simulink model "thrust_vector_rocket2_no_thrust"  (R2024b)
settings: Solver=VariableStepAuto  StartTime=0.0  StopTime=10  RelTol=1e-3
values from neighbouring files (symbols this model uses):
  A = [0 1; 0 0]    [model1_simplified.m]    (also in model2_no_thrustl.m = [0, 1, 0, 0, 0, 0; model3_thrust.m = [0, 1,      0, 0,       0, 0; model4_system_and_stability.m = jacobian(f, x))
  B = [0; -T*L/J]    [model1_simplified.m]    (also in model2_no_thrustl.m = [0; model3_thrust.m = [0   0; model4_system_and_stability.m = jacobian(f, u))
  C = [1 0]    [model1_simplified.m]    (also in model2_no_thrustl.m = [1 0 0 0 0 0; model3_thrust.m = [1 0 0 0 0 0; model4_system_and_stability.m = [1 0 0 0 0 0)
  D = 0    [model1_simplified.m]    (also in model2_no_thrustl.m = [0; 0; 0]; model3_thrust.m = [0 0; 0 0; 0 0]; model4_system_and_stability.m)
  reg = ss(A1, sys.b, sys.c, 0)    [model2_no_thrustl.m]    (also in model3_thrust.m)
  sys = ss(A,B,C,D)    [model1_simplified.m]    (also in model2_no_thrustl.m; model3_thrust.m; model4_system_and_stability.m = ss(A, B, eye(6), zeros(6,2)))
  Ts = 0.05    [model2_no_thrustl.m]    (also in model3_thrust.m; optimal_control.m; rocketParameters.mat)
  x0 = [0; 0; 0; 0; 5*pi/180; 0]    [model2_no_thrustl.m]    (also in model3_thrust.m)
libraries: slpidlib x4, mpclib x2
settings Model: Creator=wolfl  LastModifiedBy=wolfl

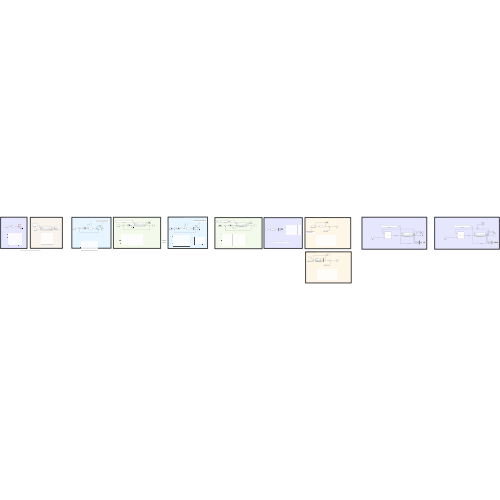
[thumbnail: Simulink's stored preview of the top-level diagram]
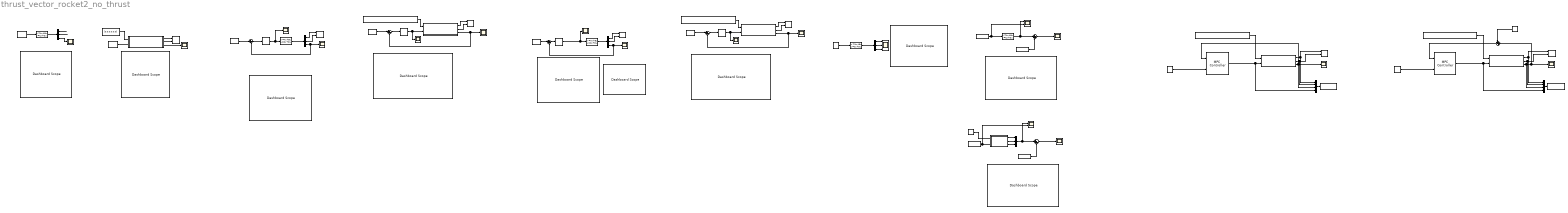
== system thrust_vector_rocket2_no_thrust ==
  note: ATTIVARE L'
      |
      | antiwindup
  note: Model Predictive Control
  note: NOTA: ricordati di selezionare "hold final value" nell'input, se no il sistema diverge malissimo!
  note: Optimal Control
  note: We can notice that this regulator allows the states to converge!
  note: Regulator with Pole Placement
  note: Non linear closed-loop
  note: Linear closed-loop
  note: Non linear open-loop
  note: Linear open-loop
  note: NOTE: We can see that in the linearized system,
      | the rocket doesn't loose altitude when it steers
  note: We can notice that the open.loop dynamic is similar only in the first few seconds.
  note: Non linear closed-loop
  note: Linear closed-loop with discrete-time controller
  note: NOTE: We can see that in the linearized system,
      | the rocket doesn't loose altitude when it steers
  note: Optimal Control - non linear system
  note: Model Predictive Control
  A+B*K : StateSpace  A=reg.a  B=reg.b  C=reg.c  D=reg.d  InitialCondition=[1,1,0,0,5*pi/180,0]
  Constant : Constant  Value=0
  Constant1 : Constant  Value=x0
  Dashboard Scope{,1..9} (10 alike) : DashboardScope
  Demux{,1..3} (4 alike) : Demux  Outputs=3
  Error : Scope
  Error1 : Scope
  Expected Output : FromWorkspace  VariableName=ySim
  Expected Output1 : FromWorkspace  VariableName=ySim
  Input from Optimal Control : FromWorkspace  VariableName=uSim  SampleTime=Ts  OutputAfterFinalValue=Holding final value
  Input from Optimal Control1 : FromWorkspace  VariableName=uSim  SampleTime=Ts  OutputAfterFinalValue=Holding final value
  MPC Controller : mpclib/MPC Controller  SCDEnableBlockLinearizationSpecification=on  mpcobj=mpc1  is_multiple=0  enable_value=0  return_u0=off  updateMPCinCallerWorkspace=on  md_inport=off  mv_inport=off  uref_inport=off  return_cost=off  return_mvseq=off  return_qpstatus=off  return_xseq=off  return_state=off  return_ovseq=off  state_inport=off  umin_inport=off  umax_inport=off  ymin_inport=off  ymax_inport=off  cc_inport=off  ywt_inport=off  uwt_inport=off  duwt_inport=off  rhoeps_inport=off  pm_inport=off  MaximumP=10  HorizonChoice=FixedHorizon  n_ts=0.05  n_p=10  n_mv=1  n_md=0  n_ud=0  n_mo=1  n_uo=0  BlockDataType=double  SampleTimeInherited=off  switch_inport=off
  MPC Controller1 : mpclib/MPC Controller  SCDEnableBlockLinearizationSpecification=on  mpcobj=mpc1  is_multiple=0  enable_value=0  return_u0=off  updateMPCinCallerWorkspace=on  md_inport=off  mv_inport=off  uref_inport=off  return_cost=off  return_mvseq=off  return_qpstatus=off  return_xseq=off  return_state=off  return_ovseq=off  state_inport=off  umin_inport=off  umax_inport=off  ymin_inport=off  ymax_inport=off  cc_inport=off  ywt_inport=off  uwt_inport=off  duwt_inport=off  rhoeps_inport=off  pm_inport=off  MaximumP=10  HorizonChoice=FixedHorizon  n_ts=0.05  n_p=10  n_mv=1  n_md=0  n_ud=0  n_mo=1  n_uo=0  BlockDataType=double  SampleTimeInherited=off  switch_inport=off
  Mux : Mux  Inputs=3
  Mux1 : Mux
  Mux2 : Mux
  Non linear System : Subsystem
  Non linear System1 : Subsystem
  Non linear System2 : Subsystem
  Non linear System3 : Subsystem
  PID Controller : slpidlib/PID Controller  Controller=PID  Form=Parallel  TimeDomain=Continuous-time  UseExternalTs=off  SampleTime=-1  IntegratorMethod=Forward Euler  FilterMethod=Forward Euler  ControllerParametersSource=internal  P=-0.206944152604434  I=-0.0701836790588113  UseKiTs=off  D=-0.149835070791128  UseExternalDerivativeSource=off  N=39.5105217733355  UseFilter=on  TunerSelectOption=Transfer Function Based (PID Tuner App)  InitialConditionSource=internal  InitialConditionForIntegrator=0  InitialConditionForFilter=0  DifferentiatorICPrevScaledInput=0  ExternalReset=none  TrackingMode=off  Kt=1  LimitOutput=on  SatLimitsSource=internal  UpperSaturationLimit=30*pi/180  LowerSaturationLimit=-30*pi/180  LinearizeAsGain=on  AntiWindupMode=none  Kb=1  LimitIntegrator=off  UpperIntegratorSaturationLimit=inf  LowerIntegratorSaturationLimit=-inf  POutMin=[]  POutMax=[]  IOutMin=[]  IOutMax=[]  DOutMin=[]  DOutMax=[]  NOutMin=[]  NOutMax=[]  SumOutMin=[]  SumOutMax=[]  SaturationOutMin=[]  SaturationOutMax=[]  PParamMin=[]  PParamMax=[]  IParamMin=[]  IParamMax=[]  DParamMin=[]  DParamMax=[]  NParamMin=[]  NParamMax=[]  KbParamMin=[]  KbParamMax=[]  KtParamMin=[]  KtParamMax=[]  KbOutMin=[]  KbOutMax=[]  KtOutMin=[]  KtOutMax=[]  IntegratorOutMin=[]  IntegratorOutMax=[]  FilterOutMin=[]  FilterOutMax=[]  SumI1OutMin=[]  SumI1OutMax=[]  SumI2OutMin=[]  SumI2OutMax=[]  SumI3OutMin=[]  SumI3OutMax=[]  SumI4OutMin=[]  SumI4OutMax=[]  SumDOutMin=[]  SumDOutMax=[]  DifferentiatorOutMin=[]  DifferentiatorOutMax=[]  FilterDiffOutCoefMin=[]  FilterDiffOutCoefMax=[]  ReciprocalOutMin=[]  ReciprocalOutMax=[]  SumDenOutMin=[]  SumDenOutMax=[]  SumNumOutMin=[]  SumNumOutMax=[]  DivideOutMin=[]  DivideOutMax=[]  UdiffTsProdOutMin=[]  UdiffTsProdOutMax=[]  NTsProdOutMin=[]  NTsProdOutMax=[]  UintegralTsProdOutMin=[]  UintegralTsProdOutMax=[]  UngainTsProdOutMin=[]  UngainTsProdOutMax=[]  ClampingZeroOutDataTypeStr=Inherit: Inherit via back propagation  ClampingZeroOutMin=[]  ClampingZeroOutMax=[]  FilterDenConstantOutDataTypeStr=Inherit: Inherit via back propagation  FilterDenConstantOutMin=[]  FilterDenConstantOutMax=[]  PCopyOutDataTypeStr=Inherit: Inherit via back propagation  PCopyOutMin=[]  PCopyOutMax=[]  NCopyOutDataTypeStr=Inherit: Inherit via back propagation  NCopyOutMin=[]  NCopyOutMax=[]  IntegratorContinuousStateAttributes=''  IntegratorStateMustResolveToSignalObject=off  IntegratorRTWStateStorageClass=Auto  FilterContinuousStateAttributes=''  FilterStateMustResolveToSignalObject=off  FilterRTWStateStorageClass=Auto  ParallelPVariant=InternalParameters  IdealPVariant=Disabled  IVariant=InternalParameters  DVariant=InternalParameters  IntegratorVariant=Continuous  SatVariant=Enabled  AWVariant=Passthrough  PCopyVariant=Disabled  TRVariant=Disabled  FdbkBlocksVariant=Forward  IdealPFdbkVariant=Disabled  SatFdbkVariant=Disabled  DerivativeFilterVariant=ContFilter  NVariant=InternalParameters  NCopyVariant=Disabled  FilterICVariant=InternalICsFilter  IntegratorICVariant=InternalICs  ExternalResetVariant=Disabled  TRSumVariant=Passthrough  SumFdbkVariant=Disabled  SumVariant=Sum_PID  TsampFilterVariant=InternalTs  TsampNgainVariant=Passthrough  TsampIntegralVariant=Disabled_SignalSpec  ExternalSaturationOutDataTypeStr=Inherit: Same as second input  DerivativeSourceVariant=ErrorSignal  PreIntVariant=InternalPreInt
  PID Controller1 : slpidlib/PID Controller  Controller=PID  Form=Parallel  TimeDomain=Continuous-time  UseExternalTs=off  SampleTime=-1  IntegratorMethod=Forward Euler  FilterMethod=Forward Euler  ControllerParametersSource=internal  P=-0.206944152604434  I=-0.0701836790588113  UseKiTs=off  D=-0.149835070791128  UseExternalDerivativeSource=off  N=39.5105217733355  UseFilter=on  TunerSelectOption=Transfer Function Based (PID Tuner App)  InitialConditionSource=internal  InitialConditionForIntegrator=0  InitialConditionForFilter=0  DifferentiatorICPrevScaledInput=0  ExternalReset=none  TrackingMode=off  Kt=1  LimitOutput=on  SatLimitsSource=internal  UpperSaturationLimit=30*pi/180  LowerSaturationLimit=-30*pi/180  LinearizeAsGain=on  AntiWindupMode=none  Kb=1  LimitIntegrator=off  UpperIntegratorSaturationLimit=inf  LowerIntegratorSaturationLimit=-inf  POutMin=[]  POutMax=[]  IOutMin=[]  IOutMax=[]  DOutMin=[]  DOutMax=[]  NOutMin=[]  NOutMax=[]  SumOutMin=[]  SumOutMax=[]  SaturationOutMin=[]  SaturationOutMax=[]  PParamMin=[]  PParamMax=[]  IParamMin=[]  IParamMax=[]  DParamMin=[]  DParamMax=[]  NParamMin=[]  NParamMax=[]  KbParamMin=[]  KbParamMax=[]  KtParamMin=[]  KtParamMax=[]  KbOutMin=[]  KbOutMax=[]  KtOutMin=[]  KtOutMax=[]  IntegratorOutMin=[]  IntegratorOutMax=[]  FilterOutMin=[]  FilterOutMax=[]  SumI1OutMin=[]  SumI1OutMax=[]  SumI2OutMin=[]  SumI2OutMax=[]  SumI3OutMin=[]  SumI3OutMax=[]  SumI4OutMin=[]  SumI4OutMax=[]  SumDOutMin=[]  SumDOutMax=[]  DifferentiatorOutMin=[]  DifferentiatorOutMax=[]  FilterDiffOutCoefMin=[]  FilterDiffOutCoefMax=[]  ReciprocalOutMin=[]  ReciprocalOutMax=[]  SumDenOutMin=[]  SumDenOutMax=[]  SumNumOutMin=[]  SumNumOutMax=[]  DivideOutMin=[]  DivideOutMax=[]  UdiffTsProdOutMin=[]  UdiffTsProdOutMax=[]  NTsProdOutMin=[]  NTsProdOutMax=[]  UintegralTsProdOutMin=[]  UintegralTsProdOutMax=[]  UngainTsProdOutMin=[]  UngainTsProdOutMax=[]  ClampingZeroOutDataTypeStr=Inherit: Inherit via back propagation  ClampingZeroOutMin=[]  ClampingZeroOutMax=[]  FilterDenConstantOutDataTypeStr=Inherit: Inherit via back propagation  FilterDenConstantOutMin=[]  FilterDenConstantOutMax=[]  PCopyOutDataTypeStr=Inherit: Inherit via back propagation  PCopyOutMin=[]  PCopyOutMax=[]  NCopyOutDataTypeStr=Inherit: Inherit via back propagation  NCopyOutMin=[]  NCopyOutMax=[]  IntegratorContinuousStateAttributes=''  IntegratorStateMustResolveToSignalObject=off  IntegratorRTWStateStorageClass=Auto  FilterContinuousStateAttributes=''  FilterStateMustResolveToSignalObject=off  FilterRTWStateStorageClass=Auto  ParallelPVariant=InternalParameters  IdealPVariant=Disabled  IVariant=InternalParameters  DVariant=InternalParameters  IntegratorVariant=Continuous  SatVariant=Enabled  AWVariant=Passthrough  PCopyVariant=Disabled  TRVariant=Disabled  FdbkBlocksVariant=Forward  IdealPFdbkVariant=Disabled  SatFdbkVariant=Disabled  DerivativeFilterVariant=ContFilter  NVariant=InternalParameters  NCopyVariant=Disabled  FilterICVariant=InternalICsFilter  IntegratorICVariant=InternalICs  ExternalResetVariant=Disabled  TRSumVariant=Passthrough  SumFdbkVariant=Disabled  SumVariant=Sum_PID  TsampFilterVariant=InternalTs  TsampNgainVariant=Passthrough  TsampIntegralVariant=Disabled_SignalSpec  ExternalSaturationOutDataTypeStr=Inherit: Same as second input  DerivativeSourceVariant=ErrorSignal  PreIntVariant=InternalPreInt
  PID Controller2 : slpidlib/PID Controller  Controller=PID  Form=Parallel  TimeDomain=Discrete-time  UseExternalTs=off  SampleTime=0.1  IntegratorMethod=Forward Euler  FilterMethod=Forward Euler  ControllerParametersSource=internal  P=-0.000166400925594158  I=-1.78058545909458e-06  UseKiTs=off  D=-0.0038876634505011  UseExternalDerivativeSource=off  N=1.14439525064094  UseFilter=off  TunerSelectOption=Transfer Function Based (PID Tuner App)  InitialConditionSource=internal  InitialConditionForIntegrator=0  InitialConditionForFilter=0  DifferentiatorICPrevScaledInput=0  ExternalReset=none  TrackingMode=off  Kt=1  LimitOutput=on  SatLimitsSource=internal  UpperSaturationLimit=30*pi/180  LowerSaturationLimit=-30*pi/180  LinearizeAsGain=on  AntiWindupMode=none  Kb=1  LimitIntegrator=off  UpperIntegratorSaturationLimit=inf  LowerIntegratorSaturationLimit=-inf  POutMin=[]  POutMax=[]  IOutMin=[]  IOutMax=[]  DOutMin=[]  DOutMax=[]  NOutMin=[]  NOutMax=[]  SumOutMin=[]  SumOutMax=[]  SaturationOutMin=[]  SaturationOutMax=[]  PParamMin=[]  PParamMax=[]  IParamMin=[]  IParamMax=[]  DParamMin=[]  DParamMax=[]  NParamMin=[]  NParamMax=[]  KbParamMin=[]  KbParamMax=[]  KtParamMin=[]  KtParamMax=[]  KbOutMin=[]  KbOutMax=[]  KtOutMin=[]  KtOutMax=[]  IntegratorOutMin=[]  IntegratorOutMax=[]  FilterOutMin=[]  FilterOutMax=[]  SumI1OutMin=[]  SumI1OutMax=[]  SumI2OutMin=[]  SumI2OutMax=[]  SumI3OutMin=[]  SumI3OutMax=[]  SumI4OutMin=[]  SumI4OutMax=[]  SumDOutMin=[]  SumDOutMax=[]  DifferentiatorOutMin=[]  DifferentiatorOutMax=[]  FilterDiffOutCoefMin=[]  FilterDiffOutCoefMax=[]  ReciprocalOutMin=[]  ReciprocalOutMax=[]  SumDenOutMin=[]  SumDenOutMax=[]  SumNumOutMin=[]  SumNumOutMax=[]  DivideOutMin=[]  DivideOutMax=[]  UdiffTsProdOutMin=[]  UdiffTsProdOutMax=[]  NTsProdOutMin=[]  NTsProdOutMax=[]  UintegralTsProdOutMin=[]  UintegralTsProdOutMax=[]  UngainTsProdOutMin=[]  UngainTsProdOutMax=[]  ClampingZeroOutDataTypeStr=Inherit: Inherit via back propagation  ClampingZeroOutMin=[]  ClampingZeroOutMax=[]  FilterDenConstantOutDataTypeStr=Inherit: Inherit via back propagation  FilterDenConstantOutMin=[]  FilterDenConstantOutMax=[]  PCopyOutDataTypeStr=Inherit: Inherit via back propagation  PCopyOutMin=[]  PCopyOutMax=[]  NCopyOutDataTypeStr=Inherit: Inherit via back propagation  NCopyOutMin=[]  NCopyOutMax=[]  IntegratorContinuousStateAttributes=''  IntegratorStateMustResolveToSignalObject=off  IntegratorRTWStateStorageClass=Auto  FilterContinuousStateAttributes=''  FilterStateMustResolveToSignalObject=off  FilterRTWStateStorageClass=Auto  ParallelPVariant=InternalParameters  IdealPVariant=Disabled  IVariant=InternalParameters  DVariant=InternalParameters  IntegratorVariant=Discrete  SatVariant=Enabled  AWVariant=Passthrough  PCopyVariant=Disabled  TRVariant=Disabled  FdbkBlocksVariant=Forward  IdealPFdbkVariant=Disabled  SatFdbkVariant=Disabled  DerivativeFilterVariant=Differentiator  NVariant=Passthrough  NCopyVariant=Disabled_SignalSpec  FilterICVariant=InternalICsDifferentiator  IntegratorICVariant=InternalICs  ExternalResetVariant=Disabled  TRSumVariant=Passthrough  SumFdbkVariant=Disabled  SumVariant=Sum_PID  TsampFilterVariant=InternalTs  TsampNgainVariant=Passthrough  TsampIntegralVariant=Disabled_SignalSpec  ExternalSaturationOutDataTypeStr=Inherit: Same as second input  DerivativeSourceVariant=ErrorSignal  PreIntVariant=InternalPreInt
  PID Controller3 : slpidlib/PID Controller  Controller=PID  Form=Parallel  TimeDomain=Continuous-time  UseExternalTs=off  SampleTime=-1  IntegratorMethod=Forward Euler  FilterMethod=Forward Euler  ControllerParametersSource=internal  P=-0.206944152604434  I=-0.0701836790588113  UseKiTs=off  D=-0.149835070791128  UseExternalDerivativeSource=off  N=39.5105217733355  UseFilter=on  TunerSelectOption=Transfer Function Based (PID Tuner App)  InitialConditionSource=internal  InitialConditionForIntegrator=0  InitialConditionForFilter=0  DifferentiatorICPrevScaledInput=0  ExternalReset=none  TrackingMode=off  Kt=1  LimitOutput=on  SatLimitsSource=internal  UpperSaturationLimit=30*pi/180  LowerSaturationLimit=-30*pi/180  LinearizeAsGain=on  AntiWindupMode=none  Kb=1  LimitIntegrator=off  UpperIntegratorSaturationLimit=inf  LowerIntegratorSaturationLimit=-inf  POutMin=[]  POutMax=[]  IOutMin=[]  IOutMax=[]  DOutMin=[]  DOutMax=[]  NOutMin=[]  NOutMax=[]  SumOutMin=[]  SumOutMax=[]  SaturationOutMin=[]  SaturationOutMax=[]  PParamMin=[]  PParamMax=[]  IParamMin=[]  IParamMax=[]  DParamMin=[]  DParamMax=[]  NParamMin=[]  NParamMax=[]  KbParamMin=[]  KbParamMax=[]  KtParamMin=[]  KtParamMax=[]  KbOutMin=[]  KbOutMax=[]  KtOutMin=[]  KtOutMax=[]  IntegratorOutMin=[]  IntegratorOutMax=[]  FilterOutMin=[]  FilterOutMax=[]  SumI1OutMin=[]  SumI1OutMax=[]  SumI2OutMin=[]  SumI2OutMax=[]  SumI3OutMin=[]  SumI3OutMax=[]  SumI4OutMin=[]  SumI4OutMax=[]  SumDOutMin=[]  SumDOutMax=[]  DifferentiatorOutMin=[]  DifferentiatorOutMax=[]  FilterDiffOutCoefMin=[]  FilterDiffOutCoefMax=[]  ReciprocalOutMin=[]  ReciprocalOutMax=[]  SumDenOutMin=[]  SumDenOutMax=[]  SumNumOutMin=[]  SumNumOutMax=[]  DivideOutMin=[]  DivideOutMax=[]  UdiffTsProdOutMin=[]  UdiffTsProdOutMax=[]  NTsProdOutMin=[]  NTsProdOutMax=[]  UintegralTsProdOutMin=[]  UintegralTsProdOutMax=[]  UngainTsProdOutMin=[]  UngainTsProdOutMax=[]  ClampingZeroOutDataTypeStr=Inherit: Inherit via back propagation  ClampingZeroOutMin=[]  ClampingZeroOutMax=[]  FilterDenConstantOutDataTypeStr=Inherit: Inherit via back propagation  FilterDenConstantOutMin=[]  FilterDenConstantOutMax=[]  PCopyOutDataTypeStr=Inherit: Inherit via back propagation  PCopyOutMin=[]  PCopyOutMax=[]  NCopyOutDataTypeStr=Inherit: Inherit via back propagation  NCopyOutMin=[]  NCopyOutMax=[]  IntegratorContinuousStateAttributes=''  IntegratorStateMustResolveToSignalObject=off  IntegratorRTWStateStorageClass=Auto  FilterContinuousStateAttributes=''  FilterStateMustResolveToSignalObject=off  FilterRTWStateStorageClass=Auto  ParallelPVariant=InternalParameters  IdealPVariant=Disabled  IVariant=InternalParameters  DVariant=InternalParameters  IntegratorVariant=Continuous  SatVariant=Enabled  AWVariant=Passthrough  PCopyVariant=Disabled  TRVariant=Disabled  FdbkBlocksVariant=Forward  IdealPFdbkVariant=Disabled  SatFdbkVariant=Disabled  DerivativeFilterVariant=ContFilter  NVariant=InternalParameters  NCopyVariant=Disabled  FilterICVariant=InternalICsFilter  IntegratorICVariant=InternalICs  ExternalResetVariant=Disabled  TRSumVariant=Passthrough  SumFdbkVariant=Disabled  SumVariant=Sum_PID  TsampFilterVariant=InternalTs  TsampNgainVariant=Passthrough  TsampIntegralVariant=Disabled_SignalSpec  ExternalSaturationOutDataTypeStr=Inherit: Same as second input  DerivativeSourceVariant=ErrorSignal  PreIntVariant=InternalPreInt
  Scope{,1..9,12,14} (12 alike) : Scope
  Scope10 : Scope  NumInputPorts=3
  Scope11 : Scope  NumInputPorts=2
  Scope13 : Scope  NumInputPorts=2
  State-Space : StateSpace  A=A  B=B  C=C  D=D  InitialCondition=[0, 0, 0, 0, 0, 0]
  State-Space1 : StateSpace  A=A  B=B  C=C  D=D  InitialCondition=[0, 0, 0, 0, 5*pi/180, 0]
  State-Space2 : StateSpace  A=A  B=B  C=C  D=D  InitialCondition=[0, 0, 0, 0, 5*pi/180, 0]
  State-Space3 : StateSpace  A=sys.a  B=sys.b  C=sys.c  D=sys.d  InitialCondition=x0
  Subsystem : Subsystem
  Subsystem1 : Subsystem
  Sum{,1..4,6} (6 alike) : Sum  Inputs=|+-
  Sum7 : Sum  Inputs=++|
  Target angle 1 : Constant  Value=0
  Target angle 2 : Constant  Value=0
  Target angle{,1..3} (4 alike) : Constant  Value=0*pi/180
  Thrust angle : Constant  Value=1*pi/180
  Thrust angle1 : Constant  Value=0*pi/180
  To Workspace : ToWorkspace  VariableName=simout1  SaveFormat=Timeseries  SampleTime=-1
  To Workspace1 : ToWorkspace  VariableName=simout  SaveFormat=Timeseries  SampleTime=-1
  White noise1 : RandomNumber  Variance=0.1*pi/180  SampleTime=0.2
  XY Graph : Record  FileSettingsInternal="{\"entries\":[{\"content\":{\"excelSettings\":{\"content\":{},\"type\":\"Streamout.ExcelSettings\"}},\"type\":\"Streamout.FileSettingStorage\",\"uuid\":\"\"}],\"packageUris\":[\"http:\\/\\/schema.mathworks.com\\/mf0\\/streamout_blocks\\/R2020a\"],\"version\":\"1.0\"}"  Layout=[1 1]  SignalsInternal="{\"entries\":[{\"content\":{\"signals\":[{\"content\":{\"blockPath\":[],\"dimensions\":[1],\"domain\":\"\",\"lineColor\":\"#fe330a\",\"lineWidth\":2,\"port\":1,\"sid\":[\"\"],\"signalID\":1,\"signalName\":\"x\"},\"type\":\"RecordBlkView.Signal\",\"uuid\":\"\"},{\"content\":{\"blockPath\":[],\"dimensions\":[1],\"domain\":\"\",\"lineColor\":\"#22b573\",\"lineWidth\":2,\"port\":2,\"sid\":[\"\"],\"signalID\":2,\"signalName\":\"y\"},\"type\":\"RecordBlkView.Signal\",\"uuid\":\"\"}]},\"type\":\"RecordBlkView.InputSignals\",\"uuid\":\"\"}],\"packageUris\":[\"http:\\/\\/schema.mathworks.com\\/mf0\\/streamout_blocks\\/R2020a\"],\"version\":\"1.0\"}"  VisualizationBindings="{\"xyplotplugin\":{\"info\":[{\"series\":[],\"subplotID\":1}]}}"  CompatibilityTag=XY
  XY Graph1 : Record  FileSettingsInternal="{\"entries\":[{\"content\":{\"excelSettings\":{\"content\":{},\"type\":\"Streamout.ExcelSettings\"}},\"type\":\"Streamout.FileSettingStorage\",\"uuid\":\"\"}],\"packageUris\":[\"http:\\/\\/schema.mathworks.com\\/mf0\\/streamout_blocks\\/R2020a\"],\"version\":\"1.0\"}"  Layout=[1 1]  SignalsInternal="{\"entries\":[{\"content\":{\"signals\":[{\"content\":{\"blockPath\":[],\"dimensions\":[1],\"domain\":\"\",\"lineColor\":\"#a2142f\",\"lineWidth\":2,\"port\":1,\"sid\":[\"\"],\"signalID\":1,\"signalName\":\"x\"},\"type\":\"RecordBlkView.Signal\",\"uuid\":\"\"},{\"content\":{\"blockPath\":[],\"dimensions\":[1],\"domain\":\"\",\"lineColor\":\"#139fff\",\"lineWidth\":2,\"port\":2,\"sid\":[\"\"],\"signalID\":2,\"signalName\":\"y\"},\"type\":\"RecordBlkView.Signal\",\"uuid\":\"\"}]},\"type\":\"RecordBlkView.InputSignals\",\"uuid\":\"\"}],\"packageUris\":[\"http:\\/\\/schema.mathworks.com\\/mf0\\/streamout_blocks\\/R2020a\"],\"version\":\"1.0\"}"  VisualizationBindings="{\"xyplotplugin\":{\"info\":[{\"series\":[],\"subplotID\":1}]}}"  CompatibilityTag=XY
  XY Graph2 : Record  FileSettingsInternal="{\"entries\":[{\"content\":{\"excelSettings\":{\"content\":{},\"type\":\"Streamout.ExcelSettings\"}},\"type\":\"Streamout.FileSettingStorage\",\"uuid\":\"\"}],\"packageUris\":[\"http:\\/\\/schema.mathworks.com\\/mf0\\/streamout_blocks\\/R2020a\"],\"version\":\"1.0\"}"  Layout=[1 1]  SignalsInternal="{\"entries\":[{\"content\":{\"signals\":[{\"content\":{\"blockPath\":[],\"dimensions\":[1],\"domain\":\"\",\"lineColor\":\"#64d413\",\"lineWidth\":2,\"port\":1,\"sid\":[\"\"],\"signalID\":1,\"signalName\":\"x\"},\"type\":\"RecordBlkView.Signal\",\"uuid\":\"\"},{\"content\":{\"blockPath\":[],\"dimensions\":[1],\"domain\":\"\",\"lineColor\":\"#ff13a6\",\"lineWidth\":2,\"port\":2,\"sid\":[\"\"],\"signalID\":2,\"signalName\":\"y\"},\"type\":\"RecordBlkView.Signal\",\"uuid\":\"\"}]},\"type\":\"RecordBlkView.InputSignals\",\"uuid\":\"\"}],\"packageUris\":[\"http:\\/\\/schema.mathworks.com\\/mf0\\/streamout_blocks\\/R2020a\"],\"version\":\"1.0\"}"  VisualizationBindings="{\"xyplotplugin\":{\"info\":[{\"series\":[],\"subplotID\":1}]}}"  CompatibilityTag=XY
  XY Graph3 : Record  FileSettingsInternal="{\"entries\":[{\"content\":{\"excelSettings\":{\"content\":{},\"type\":\"Streamout.ExcelSettings\"}},\"type\":\"Streamout.FileSettingStorage\",\"uuid\":\"\"}],\"packageUris\":[\"http:\\/\\/schema.mathworks.com\\/mf0\\/streamout_blocks\\/R2020a\"],\"version\":\"1.0\"}"  Layout=[1 1]  SignalsInternal="{\"entries\":[{\"content\":{\"signals\":[{\"content\":{\"blockPath\":[],\"dimensions\":[1],\"domain\":\"\",\"lineColor\":\"#ff6929\",\"lineWidth\":2,\"port\":1,\"sid\":[\"\"],\"signalID\":1,\"signalName\":\"x\"},\"type\":\"RecordBlkView.Signal\",\"uuid\":\"\"},{\"content\":{\"blockPath\":[],\"dimensions\":[1],\"domain\":\"\",\"lineColor\":\"#b746ff\",\"lineWidth\":2,\"port\":2,\"sid\":[\"\"],\"signalID\":2,\"signalName\":\"y\"},\"type\":\"RecordBlkView.Signal\",\"uuid\":\"\"}]},\"type\":\"RecordBlkView.InputSignals\",\"uuid\":\"\"}],\"packageUris\":[\"http:\\/\\/schema.mathworks.com\\/mf0\\/streamout_blocks\\/R2020a\"],\"version\":\"1.0\"}"  VisualizationBindings="{\"xyplotplugin\":{\"info\":[{\"series\":[],\"subplotID\":1}]}}"  CompatibilityTag=XY
  XY Graph4 : Record  FileSettingsInternal="{\"entries\":[{\"content\":{\"excelSettings\":{\"content\":{},\"type\":\"Streamout.ExcelSettings\"}},\"type\":\"Streamout.FileSettingStorage\",\"uuid\":\"\"}],\"packageUris\":[\"http:\\/\\/schema.mathworks.com\\/mf0\\/streamout_blocks\\/R2020a\"],\"version\":\"1.0\"}"  Layout=[1 1]  SignalsInternal="{\"entries\":[{\"content\":{\"signals\":[{\"content\":{\"blockPath\":[],\"dimensions\":[1],\"domain\":\"\",\"lineColor\":\"#a2142f\",\"plots\":[ 1 ],\"port\":1,\"sid\":[\"\"],\"signalID\":1,\"signalName\":\"x\"},\"type\":\"RecordBlkView.Signal\",\"uuid\":\"\"},{\"content\":{\"blockPath\":[],\"dimensions\":[1],\"domain\":\"\",\"lineColor\":\"#139fff\",\"plots\":[ 1 ],\"port\":2,\"sid\":[\"\"],\"signalID\":2,\"signalName\":\"y\"},\"type\":\"RecordBlkView.Signal\",\"uuid\":\"\"}]},\"type\":\"RecordBlkView.InputSignals\",\"uuid\":\"\"}],\"packageUris\":[\"http:\\/\\/schema.mathworks.com\\/mf0\\/streamout_blocks\\/R2020a\"],\"version\":\"1.0\"}"  VisualizationBindings="{\"xyplotplugin\":{\"info\":[{\"series\":[{\"bindingParametersList\":[{\"parameter\":\"X-Axis\",\"signalID\":1,\"signalName\":\"x\"},{\"parameter\":\"Y-Axis\",\"signalID\":2,\"signalName\":\"y\"}],\"seriesID\":0}],\"subplotID\":1}]}}"  CompatibilityTag=XY
  XY Graph5 : Record  FileSettingsInternal="{\"entries\":[{\"content\":{\"excelSettings\":{\"content\":{},\"type\":\"Streamout.ExcelSettings\"}},\"type\":\"Streamout.FileSettingStorage\",\"uuid\":\"\"}],\"packageUris\":[\"http:\\/\\/schema.mathworks.com\\/mf0\\/streamout_blocks\\/R2020a\"],\"version\":\"1.0\"}"  Layout=[1 1]  SignalsInternal="{\"entries\":[{\"content\":{\"signals\":[{\"content\":{\"blockPath\":[],\"dimensions\":[1],\"domain\":\"\",\"lineColor\":\"#a2142f\",\"plots\":[ 1 ],\"port\":1,\"sid\":[\"\"],\"signalID\":1,\"signalName\":\"x\"},\"type\":\"RecordBlkView.Signal\",\"uuid\":\"\"},{\"content\":{\"blockPath\":[],\"dimensions\":[1],\"domain\":\"\",\"lineColor\":\"#139fff\",\"plots\":[ 1 ],\"port\":2,\"sid\":[\"\"],\"signalID\":2,\"signalName\":\"y\"},\"type\":\"RecordBlkView.Signal\",\"uuid\":\"\"}]},\"type\":\"RecordBlkView.InputSignals\",\"uuid\":\"\"}],\"packageUris\":[\"http:\\/\\/schema.mathworks.com\\/mf0\\/streamout_blocks\\/R2020a\"],\"version\":\"1.0\"}"  VisualizationBindings="{\"xyplotplugin\":{\"info\":[{\"series\":[{\"bindingParametersList\":[{\"parameter\":\"X-Axis\",\"signalID\":1,\"signalName\":\"x\"},{\"parameter\":\"Y-Axis\",\"signalID\":2,\"signalName\":\"y\"}],\"seriesID\":0}],\"subplotID\":1}]}}"  CompatibilityTag=XY
  XY Graph6 : Record  FileSettingsInternal="{\"entries\":[{\"content\":{\"excelSettings\":{\"content\":{},\"type\":\"Streamout.ExcelSettings\"}},\"type\":\"Streamout.FileSettingStorage\",\"uuid\":\"\"}],\"packageUris\":[\"http:\\/\\/schema.mathworks.com\\/mf0\\/streamout_blocks\\/R2020a\"],\"version\":\"1.0\"}"  Layout=[1 1]  SignalsInternal="{\"entries\":[{\"content\":{\"signals\":[{\"content\":{\"blockPath\":[],\"dimensions\":[1],\"domain\":\"\",\"lineColor\":\"#a2142f\",\"plots\":[ 1 ],\"port\":1,\"signalID\":1,\"signalName\":\"x\"},\"type\":\"RecordBlkView.Signal\",\"uuid\":\"\"},{\"content\":{\"blockPath\":[],\"dimensions\":[1],\"domain\":\"\",\"lineColor\":\"#139fff\",\"plots\":[ 1 ],\"port\":2,\"signalID\":2,\"signalName\":\"y\"},\"type\":\"RecordBlkView.Signal\",\"uuid\":\"\"}]},\"type\":\"RecordBlkView.InputSignals\",\"uuid\":\"\"}],\"packageUris\":[\"http:\\/\\/schema.mathworks.com\\/mf0\\/streamout_blocks\\/R2020a\"],\"version\":\"1.0\"}"  VisualizationBindings="{\"xyplotplugin\":{\"info\":[{\"series\":[{\"bindingParametersList\":[{\"parameter\":\"X-Axis\",\"signalID\":1,\"signalName\":\"x\"},{\"parameter\":\"Y-Axis\",\"signalID\":2,\"signalName\":\"y\"}],\"seriesID\":0}],\"subplotID\":1}]}}"  CompatibilityTag=XY
  initial state : Constant  Value=[0,0,0,0,0,0]
  initial state{1..4} (4 alike) : Constant  Value=[0,0,0,0,5*pi/180,0]
  wires:
  Thrust angle/1 -> State-Space/1
  State-Space/1 -> Demux/1
  Thrust angle1/1 -> Subsystem/2(thrust angle)
  initial state/1 -> Subsystem/1(initial state)
  Subsystem/3(theta) -> Scope1/1  "rocket angle"
  Subsystem/1(Output) -> XY Graph5/1  "x"
  Subsystem/2(Output1) -> XY Graph5/2  "y"
  Demux/1 -> ?  "x"
  Demux/3 -> Scope/1  "theta"
  Demux/2 -> ?  "y"
  Demux1/2 -> XY Graph1/2  "y"
  Demux1/1 -> XY Graph1/1  "x"
  State-Space1/1 -> Demux1/1
  Demux1/3 -> Sum/2, Scope2/1  "theta"
  Target angle/1 -> Sum/1
  Sum/1 -> PID Controller/1
  PID Controller/1 -> Scope3/1, State-Space1/1  "phi"
  Target angle1/1 -> Sum1/1
  Sum1/1 -> PID Controller1/1
  PID Controller1/1 -> Subsystem1/2(thrust angle), Scope5/1  "phi"
  Subsystem1/3(theta) -> Scope4/1, Sum1/2  "theta"
  Subsystem1/2(Output1) -> XY Graph/2  "y"
  Subsystem1/1(Output) -> XY Graph/1  "x"
  initial state1/1 -> Subsystem1/1(initial state)
  initial state2/1 -> Non linear System/1(initial state)
  Target angle3/1 -> Sum3/1
  PID Controller3/1 -> Non linear System/2(thrust angle), Scope9/1  "phi"
  Non linear System/3(theta) -> Scope8/1, Sum3/2  "theta"
  Target angle2/1 -> Sum2/1
  Sum2/1 -> PID Controller2/1
  Demux2/1 -> XY Graph3/1  "x"
  PID Controller2/1 -> Scope7/1, State-Space2/1  "phi"
  Sum3/1 -> PID Controller3/1
  State-Space2/1 -> Demux2/1
  Demux2/3 -> Sum2/2, Scope6/1  "theta"
  Non linear System/1(Output) -> XY Graph2/1  "x"
  Demux2/2 -> XY Graph3/2  "y"
  Non linear System/2(Output1) -> XY Graph2/2  "y"
  A+B*K/1 -> Demux3/1
  Constant/1 -> A+B*K/1
  Demux3/1 -> Scope10/1  "x"
  Demux3/2 -> Scope10/2  "y"
  Demux3/3 -> Scope10/3  "theta"
  Input from Optimal Control/1 -> State-Space3/1, Scope11/2  "u"
  State-Space3/1 -> Scope11/1, Sum4/1  "output"
  Expected Output/1 -> Sum4/2
  Sum4/1 -> Error/1
  MPC Controller/1 -> Mux1/4, Non linear System1/2(thrust angle)  "thrust angle"
  initial state3/1 -> Non linear System1/1(initial state)
  Target angle 2/1 -> MPC Controller/2
  Mux1/1 -> To Workspace/1
  Non linear System1/2(y) -> Mux1/2, XY Graph4/2  "y"
  Non linear System1/1(x) -> Mux1/1, XY Graph4/1  "x"
  Non linear System1/3(theta) -> MPC Controller/1, Scope12/1, Mux1/3  "theta"
  Sum6/1 -> Error1/1
  Expected Output1/1 -> Sum6/2
  Input from Optimal Control1/1 -> Scope13/2, Non linear System2/2(thrust angle)  "u"
  Mux/1 -> Sum6/1, Scope13/1  "output"
  Non linear System2/1(Output) -> Mux/1  "x"
  Non linear System2/2(Output1) -> Mux/2  "y"
  Non linear System2/3(theta) -> Mux/3  "theta"
  Constant1/1 -> Non linear System2/1(initial state)
  initial state4/1 -> Non linear System3/1(initial state)
  Non linear System3/1(x) -> Mux2/1, XY Graph6/1  "x"
  Non linear System3/3(theta) -> Mux2/3, Scope14/1, Sum7/2  "theta"
  Non linear System3/2(y) -> Mux2/2, XY Graph6/2  "y"
  Sum7/1 -> MPC Controller1/1
  Mux2/1 -> To Workspace1/1
  White noise1/1 -> Sum7/1
  MPC Controller1/1 -> Mux2/4, Non linear System3/2(thrust angle)  "thrust angle"
  Target angle 1/1 -> MPC Controller1/2

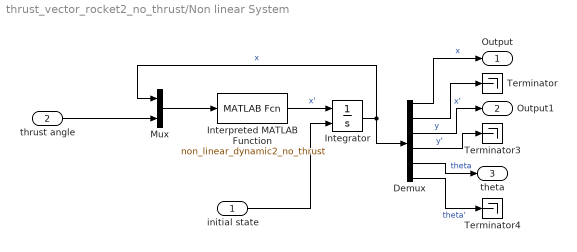
== system thrust_vector_rocket2_no_thrust/Non linear System ==
  initial state : Inport
  thrust angle : Inport  Port=2
  Demux : Demux  Outputs=6
  Integrator : Integrator  InitialConditionSource=external
  Interpreted MATLAB Function : MATLABFcn  MATLABFcn=non_linear_dynamic2_no_thrust
  Mux : Mux  Inputs=2
  Terminator : Terminator
  Terminator3 : Terminator
  Terminator4 : Terminator
  Output : Outport
  Output1 : Outport  Port=2
  theta : Outport  Port=3
  wires:
  thrust angle/1 -> Mux/2
  Interpreted MATLAB Function/1 -> Integrator/1  "x'"
  Mux/1 -> Interpreted MATLAB Function/1
  Demux/1 -> Output/1  "x"
  Demux/2 -> Terminator/1  "x'"
  Integrator/1 -> Mux/1, Demux/1  "x"
  initial state/1 -> Integrator/2
  Demux/3 -> Output1/1  "y"
  Demux/4 -> Terminator3/1  "y'"
  Demux/5 -> theta/1  "theta"
  Demux/6 -> Terminator4/1  "theta'"

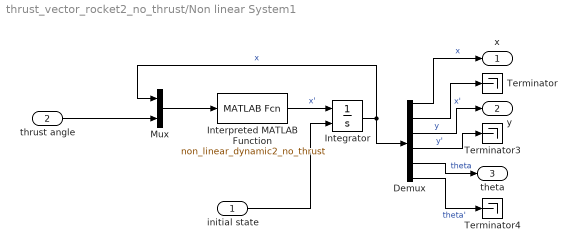
== system thrust_vector_rocket2_no_thrust/Non linear System1 ==
  initial state : Inport
  thrust angle : Inport  Port=2
  Demux : Demux  Outputs=6
  Integrator : Integrator  InitialConditionSource=external
  Interpreted MATLAB Function : MATLABFcn  MATLABFcn=non_linear_dynamic2_no_thrust
  Mux : Mux  Inputs=2
  Terminator : Terminator
  Terminator3 : Terminator
  Terminator4 : Terminator
  x : Outport
  y : Outport  Port=2
  theta : Outport  Port=3
  wires:
  thrust angle/1 -> Mux/2
  Interpreted MATLAB Function/1 -> Integrator/1  "x'"
  Mux/1 -> Interpreted MATLAB Function/1
  Demux/1 -> x/1  "x"
  Demux/2 -> Terminator/1  "x'"
  Integrator/1 -> Mux/1, Demux/1  "x"
  initial state/1 -> Integrator/2
  Demux/3 -> y/1  "y"
  Demux/4 -> Terminator3/1  "y'"
  Demux/5 -> theta/1  "theta"
  Demux/6 -> Terminator4/1  "theta'"

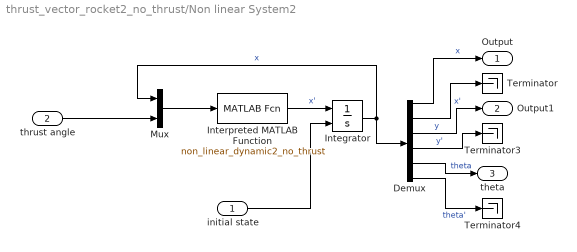
== system thrust_vector_rocket2_no_thrust/Non linear System2 ==
  initial state : Inport
  thrust angle : Inport  Port=2
  Demux : Demux  Outputs=6
  Integrator : Integrator  InitialConditionSource=external
  Interpreted MATLAB Function : MATLABFcn  MATLABFcn=non_linear_dynamic2_no_thrust
  Mux : Mux  Inputs=2
  Terminator : Terminator
  Terminator3 : Terminator
  Terminator4 : Terminator
  Output : Outport
  Output1 : Outport  Port=2
  theta : Outport  Port=3
  wires:
  thrust angle/1 -> Mux/2
  Interpreted MATLAB Function/1 -> Integrator/1  "x'"
  Mux/1 -> Interpreted MATLAB Function/1
  Demux/1 -> Output/1  "x"
  Demux/2 -> Terminator/1  "x'"
  Integrator/1 -> Mux/1, Demux/1  "x"
  initial state/1 -> Integrator/2
  Demux/3 -> Output1/1  "y"
  Demux/4 -> Terminator3/1  "y'"
  Demux/5 -> theta/1  "theta"
  Demux/6 -> Terminator4/1  "theta'"

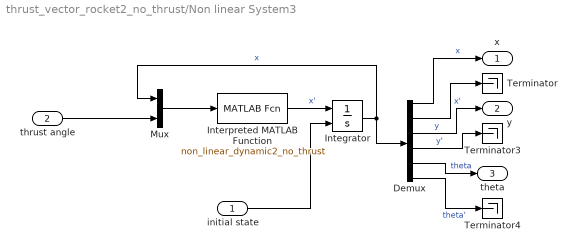
== system thrust_vector_rocket2_no_thrust/Non linear System3 ==
  initial state : Inport
  thrust angle : Inport  Port=2
  Demux : Demux  Outputs=6
  Integrator : Integrator  InitialConditionSource=external
  Interpreted MATLAB Function : MATLABFcn  MATLABFcn=non_linear_dynamic2_no_thrust
  Mux : Mux  Inputs=2
  Terminator : Terminator
  Terminator3 : Terminator
  Terminator4 : Terminator
  x : Outport
  y : Outport  Port=2
  theta : Outport  Port=3
  wires:
  thrust angle/1 -> Mux/2
  Interpreted MATLAB Function/1 -> Integrator/1  "x'"
  Mux/1 -> Interpreted MATLAB Function/1
  Demux/1 -> x/1  "x"
  Demux/2 -> Terminator/1  "x'"
  Integrator/1 -> Mux/1, Demux/1  "x"
  initial state/1 -> Integrator/2
  Demux/3 -> y/1  "y"
  Demux/4 -> Terminator3/1  "y'"
  Demux/5 -> theta/1  "theta"
  Demux/6 -> Terminator4/1  "theta'"

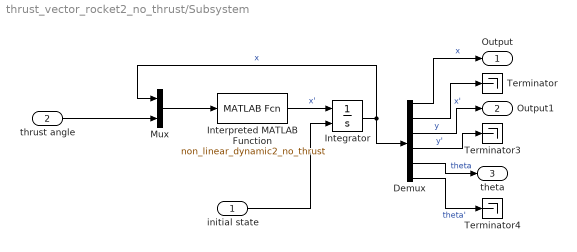
== system thrust_vector_rocket2_no_thrust/Subsystem ==
  initial state : Inport
  thrust angle : Inport  Port=2
  Demux : Demux  Outputs=6
  Integrator : Integrator  InitialConditionSource=external
  Interpreted MATLAB Function : MATLABFcn  MATLABFcn=non_linear_dynamic2_no_thrust
  Mux : Mux  Inputs=2
  Terminator : Terminator
  Terminator3 : Terminator
  Terminator4 : Terminator
  Output : Outport
  Output1 : Outport  Port=2
  theta : Outport  Port=3
  wires:
  thrust angle/1 -> Mux/2
  Interpreted MATLAB Function/1 -> Integrator/1  "x'"
  Mux/1 -> Interpreted MATLAB Function/1
  Demux/1 -> Output/1  "x"
  Demux/2 -> Terminator/1  "x'"
  Integrator/1 -> Mux/1, Demux/1  "x"
  initial state/1 -> Integrator/2
  Demux/3 -> Output1/1  "y"
  Demux/4 -> Terminator3/1  "y'"
  Demux/5 -> theta/1  "theta"
  Demux/6 -> Terminator4/1  "theta'"

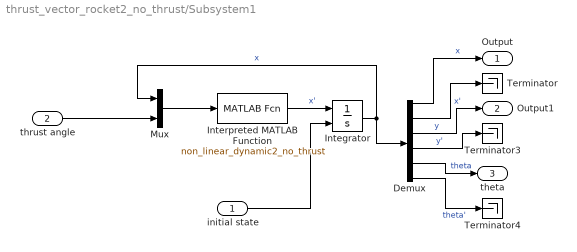
== system thrust_vector_rocket2_no_thrust/Subsystem1 ==
  initial state : Inport
  thrust angle : Inport  Port=2
  Demux : Demux  Outputs=6
  Integrator : Integrator  InitialConditionSource=external
  Interpreted MATLAB Function : MATLABFcn  MATLABFcn=non_linear_dynamic2_no_thrust
  Mux : Mux  Inputs=2
  Terminator : Terminator
  Terminator3 : Terminator
  Terminator4 : Terminator
  Output : Outport
  Output1 : Outport  Port=2
  theta : Outport  Port=3
  wires:
  thrust angle/1 -> Mux/2
  Interpreted MATLAB Function/1 -> Integrator/1  "x'"
  Mux/1 -> Interpreted MATLAB Function/1
  Demux/1 -> Output/1  "x"
  Demux/2 -> Terminator/1  "x'"
  Integrator/1 -> Mux/1, Demux/1  "x"
  initial state/1 -> Integrator/2
  Demux/3 -> Output1/1  "y"
  Demux/4 -> Terminator3/1  "y'"
  Demux/5 -> theta/1  "theta"
  Demux/6 -> Terminator4/1  "theta'"
